simulink model "hps_projekat"  (R2024a)
settings: Solver=VariableStepAuto  StartTime=0.0  StopTime=30  RelTol=1e-3
values from neighbouring files (symbols this model uses):
  a21 = -(k+K)/(Mt+10*m/3)    (= -2377.17908082)    [inic_param.m]
  a22 = -(Bp + b)/(Mt+10*m/3)    (= -0.332805071315)    [inic_param.m]
  a23 = (k)/(Mt+10*m/3)    (= 2377.17908082)    [inic_param.m]
  a24 = b/(Mt+10*m/3)    (= 0.297147385103)    [inic_param.m]
  a25 = Ap/(Mt+10*m/3)    (= 3.56576862124e-06)    [inic_param.m]
  a41 = k/(3*m)    (= 2666.66666667)    [inic_param.m]
  a42 = b/(3*m)    (= 0.333333333333)    [inic_param.m]
  a43 = -k/(3*m)    (= -2666.66666667)    [inic_param.m]
  a44 = -b/(3*m)    (= -0.333333333333)    [inic_param.m]
  a52 = -4*Ap*Be/Vt    (= -3900000000)    [inic_param.m]
  a55 = -(Ctp+Kc)*4*Be/Vt    (= -2.587)    [inic_param.m]
  Ap = 3 * 10^(-3)    (= 0.003)    [inic_param.m]
  b5 = Kt*Kq*4*Be/ (r_pov_opruge*R*Kf*Vt)    (= 3567200000)    [inic_param.m]
  Bp = 30    [inic_param.m]
  F = 500    [inic_param.m]
  h4 = -1/(3*m)    (= -0.00133333333333)    [inic_param.m]
  K = 0    [inic_param.m]
  Mt = 8    [inic_param.m]
libraries: slpidlib x1
settings Model: Creator=Korisnik  LastModifiedBy=Korisnik

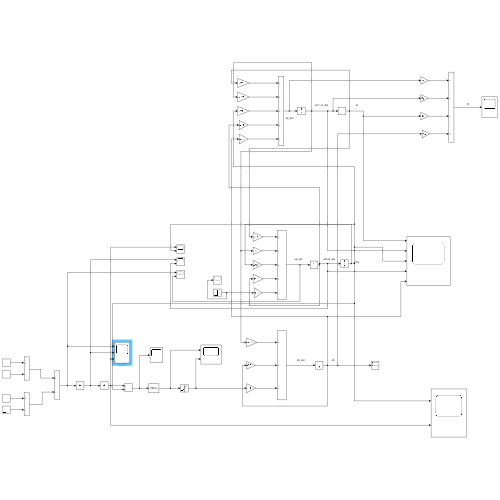
[thumbnail: Simulink's stored preview of the top-level diagram]
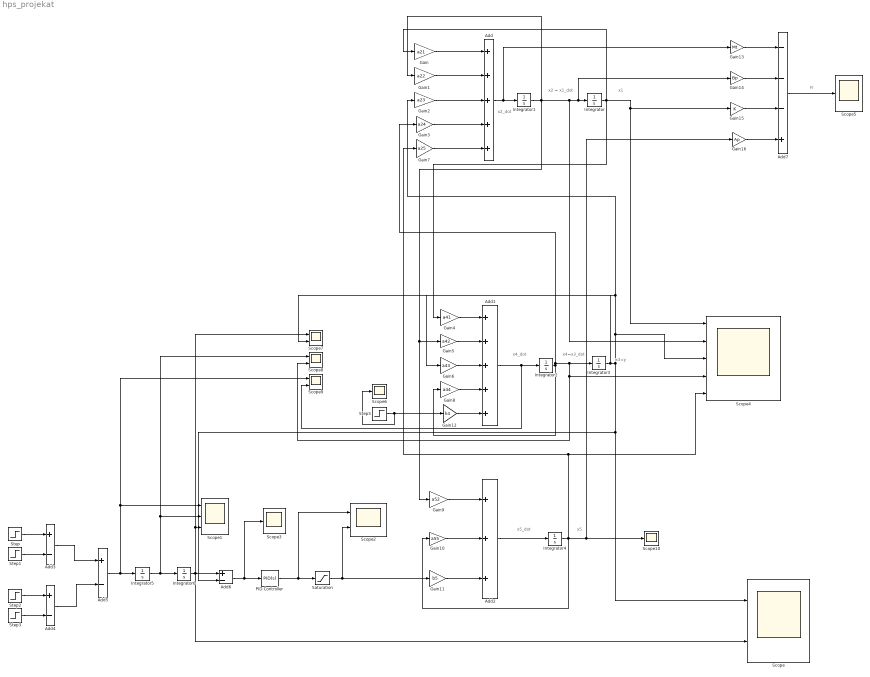
== system hps_projekat ==
  note: Fl
  note: x5_dot
  note: x4=x3_dot
  note: x2_dot
  note: x5
  note: x4_dot
  note: x3=y
  note: x1
  note: x2 = x1_dot
  Add : Sum  Inputs=+++++
  Add1 : Sum  Inputs=+++++
  Add2 : Sum  Inputs=+++
  Add{3..6} (4 alike) : Sum  Inputs=+-
  Add7 : Sum  Inputs=---+
  Gain : Gain  Gain=a21
  Gain1 : Gain  Gain=a22
  Gain10 : Gain  Gain=a55
  Gain11 : Gain  Gain=b5
  Gain12 : Gain  Gain=h4
  Gain13 : Gain  Gain=Mt
  Gain14 : Gain  Gain=Bp
  Gain15 : Gain  Gain=K
  Gain16 : Gain  Gain=Ap
  Gain2 : Gain  Gain=a23
  Gain3 : Gain  Gain=a24
  Gain4 : Gain  Gain=a41
  Gain5 : Gain  Gain=a42
  Gain6 : Gain  Gain=a43
  Gain7 : Gain  Gain=a25
  Gain8 : Gain  Gain=a44
  Gain9 : Gain  Gain=a52
  Integrator{,1..6} (7 alike) : Integrator
  PID Controller : slpidlib/PID Controller  Controller=PID  Form=Parallel  TimeDomain=Continuous-time  UseExternalTs=off  SampleTime=-1  IntegratorMethod=Forward Euler  FilterMethod=Forward Euler  ControllerParametersSource=internal  P=0.69*0.6  I=0.69*0.6*2/0.1335  UseKiTs=off  D=0.69*0.6*0.1335/8  UseExternalDerivativeSource=off  N=100  UseFilter=on  TunerSelectOption=Transfer Function Based (PID Tuner App)  InitialConditionSource=internal  InitialConditionForIntegrator=0  InitialConditionForFilter=0  DifferentiatorICPrevScaledInput=0  ExternalReset=none  TrackingMode=off  Kt=1  LimitOutput=off  SatLimitsSource=internal  UpperSaturationLimit=inf  LowerSaturationLimit=-inf  LinearizeAsGain=on  AntiWindupMode=none  Kb=1  LimitIntegrator=off  UpperIntegratorSaturationLimit=inf  LowerIntegratorSaturationLimit=-inf  POutMin=[]  POutMax=[]  IOutMin=[]  IOutMax=[]  DOutMin=[]  DOutMax=[]  NOutMin=[]  NOutMax=[]  SumOutMin=[]  SumOutMax=[]  SaturationOutMin=[]  SaturationOutMax=[]  PParamMin=[]  PParamMax=[]  IParamMin=[]  IParamMax=[]  DParamMin=[]  DParamMax=[]  NParamMin=[]  NParamMax=[]  KbParamMin=[]  KbParamMax=[]  KtParamMin=[]  KtParamMax=[]  KbOutMin=[]  KbOutMax=[]  KtOutMin=[]  KtOutMax=[]  IntegratorOutMin=[]  IntegratorOutMax=[]  FilterOutMin=[]  FilterOutMax=[]  SumI1OutMin=[]  SumI1OutMax=[]  SumI2OutMin=[]  SumI2OutMax=[]  SumI3OutMin=[]  SumI3OutMax=[]  SumI4OutMin=[]  SumI4OutMax=[]  SumDOutMin=[]  SumDOutMax=[]  DifferentiatorOutMin=[]  DifferentiatorOutMax=[]  FilterDiffOutCoefMin=[]  FilterDiffOutCoefMax=[]  ReciprocalOutMin=[]  ReciprocalOutMax=[]  SumDenOutMin=[]  SumDenOutMax=[]  SumNumOutMin=[]  SumNumOutMax=[]  DivideOutMin=[]  DivideOutMax=[]  UdiffTsProdOutMin=[]  UdiffTsProdOutMax=[]  NTsProdOutMin=[]  NTsProdOutMax=[]  UintegralTsProdOutMin=[]  UintegralTsProdOutMax=[]  UngainTsProdOutMin=[]  UngainTsProdOutMax=[]  ClampingZeroOutDataTypeStr=Inherit: Inherit via back propagation  ClampingZeroOutMin=[]  ClampingZeroOutMax=[]  FilterDenConstantOutDataTypeStr=Inherit: Inherit via back propagation  FilterDenConstantOutMin=[]  FilterDenConstantOutMax=[]  PCopyOutDataTypeStr=Inherit: Inherit via back propagation  PCopyOutMin=[]  PCopyOutMax=[]  NCopyOutDataTypeStr=Inherit: Inherit via back propagation  NCopyOutMin=[]  NCopyOutMax=[]  IntegratorContinuousStateAttributes=''  IntegratorStateMustResolveToSignalObject=off  IntegratorRTWStateStorageClass=Auto  FilterContinuousStateAttributes=''  FilterStateMustResolveToSignalObject=off  FilterRTWStateStorageClass=Auto  ParallelPVariant=InternalParameters  IdealPVariant=Disabled  IVariant=InternalParameters  DVariant=InternalParameters  IntegratorVariant=Continuous  SatVariant=Disabled  AWVariant=Passthrough  PCopyVariant=Disabled  TRVariant=Disabled  FdbkBlocksVariant=Forward  IdealPFdbkVariant=Disabled  SatFdbkVariant=Disabled  DerivativeFilterVariant=ContFilter  NVariant=InternalParameters  NCopyVariant=Disabled  FilterICVariant=InternalICsFilter  IntegratorICVariant=InternalICs  ExternalResetVariant=Disabled  TRSumVariant=Passthrough  SumFdbkVariant=Disabled  SumVariant=Sum_PID  TsampFilterVariant=InternalTs  TsampNgainVariant=Passthrough  TsampIntegralVariant=Disabled_SignalSpec  ExternalSaturationOutDataTypeStr=Inherit: Same as second input  DerivativeSourceVariant=ErrorSignal
  Saturation : Saturate  UpperLimit=24  LowerLimit=-24
  Scope{,2,7..9} (5 alike) : Scope  NumInputPorts=2
  Scope1 : Scope  NumInputPorts=3
  Scope{3,5..6,10} (4 alike) : Scope
  Scope4 : Scope  NumInputPorts=5
  Step : Step  After=1.5686  SampleTime=0
  Step1 : Step  Time=1.45  After=1.5686  SampleTime=0
  Step2 : Step  Time=3.55  After=1.5686  SampleTime=0
  Step3 : Step  Time=4  After=1.5686  SampleTime=0
  Step5 : Step  After=F  SampleTime=0
  wires:
  Integrator3/1 -> Scope7/2, Add6/2, Scope/1, Gain6/1, Gain2/1, Scope4/3
  Gain11/1 -> Add2/3
  Add2/1 -> Integrator4/1
  Integrator2/1 -> Gain3/1, Scope8/2, Scope4/4, Integrator3/1, Gain8/1
  Integrator4/1 -> Scope10/1, Gain16/1, Scope4/5, Gain7/1, Gain10/1
  Gain8/1 -> Add1/4
  Gain3/1 -> Add/4
  Gain7/1 -> Add/5
  Gain/1 -> Add/1
  Gain5/1 -> Add1/2
  Add/1 -> Integrator1/1, Gain13/1
  Gain2/1 -> Add/3
  Integrator/1 -> Gain/1, Gain15/1, Scope4/1, Gain4/1
  Gain10/1 -> Add2/2
  Gain4/1 -> Add1/1
  Integrator1/1 -> Gain9/1, Gain5/1, Gain1/1, Gain14/1, Integrator/1, Scope4/2
  Add1/1 -> Scope9/2, Integrator2/1
  Gain9/1 -> Add2/1
  Gain6/1 -> Add1/3
  Gain1/1 -> Add/2
  Integrator6/1 -> Scope/2, Scope7/1, Scope1/3, Add6/1
  Step3/1 -> Add4/2
  Integrator5/1 -> Scope8/1, Scope1/2, Integrator6/1
  Add4/1 -> Add5/2
  Add3/1 -> Add5/1
  Step/1 -> Add3/1
  Add5/1 -> Scope9/1, Scope1/1, Integrator5/1
  Step1/1 -> Add3/2
  Step2/1 -> Add4/1
  Add6/1 -> PID Controller/1, Scope3/1
  Saturation/1 -> Gain11/1, Scope2/2
  Gain12/1 -> Add1/5
  Step5/1 -> Scope6/1, Gain12/1
  Gain16/1 -> Add7/4
  Gain15/1 -> Add7/3
  Gain14/1 -> Add7/2
  Gain13/1 -> Add7/1
  Add7/1 -> Scope5/1
  PID Controller/1 -> Scope2/1, Saturation/1
